simulink model "model"  (R2021a)
settings: Solver=VariableStepDiscrete  StartTime=0.0  StopTime=1000  RelTol=1e-3  EnableMultiTasking=on
PreLoadFcn:
  | initmod
values from neighbouring files (symbols this model uses):
  Bit_pat = Create_pat([1,0],1/(Ftr*2)-1/(2*Frc),1/Frc)    [initmod.m]
  Frc = Ftr*k    (= 16000)    [initmod.m]
  Ftr = 2000    [initmod.m]
  k = k+1    (= 2)    [initmod.m]
  pack_len = 11    [initmod.m]
  Preamble = [1,1,0,1,1,0,0,1,1,1,0,0,0,0,1,0]    [initmod.m]
  Preamble_decis_levl = ((Preamble_pat_len-Manchester_crosscorrelation*k/2)/2+Preamble_pat_len/2+Preamble_pat_len)/2-3    [initmod.m]
  Preamble_pat = Create_pat(Preamble,1/(Ftr*2),1/Frc)    [initmod.m]
  Preamble_pat_len = length(Preamble_pat)    [initmod.m]
undefined symbols (not defined in the file or in its folder): Bit_pat_len
libraries: dspobslib x14, dspswit3 x9, dspsigops x5, commutil2 x4, dspindex x4, commrandsrc3 x2, simulink_extras x1, commrandsrc2 x1, dspstat3 x1, commsink2 x1
settings Model: Creator=DeveloperY  LastModifiedBy=DeveloperY
settings DataIOCC: InitialState=init  LimitDataPoints=on  SaveFormat=Array  SignalLoggingSaveFormat=ModelDataLogs  ReturnWorkspaceOutputs=off
settings OptimizationCC: BlockReduction=off  BooleanDataType=off  OptimizeBlockIOStorage=off  BufferReuse=off  ExpressionFolding=off  LocalBlockOutputs=off  InitFltsAndDblsToZero=on  LifeSpan=inf
settings DebuggingCC: SaveWithParameterizedLinksMsg=none  UnderspecifiedInitializationDetection=Classic  MergeDetectMultiDrivingBlocksExec=none  SignalResolutionControl=TryResolveAllWithWarning  MultiTaskDSMMsg=warning  MultiTaskCondExecSysMsg=none  FcnCallInpInsideContextMsg=warning  SFUnexpectedBacktrackingDiag=warning  SFNoUnconditionalDefaultTransitionDiag=warning  SFExecutionAtInitializationDiag=none  SFMachineParentedDataDiag=warning  ArithmeticOperatorsInVariantConditions=warning
settings HardwareCC: ProdBitPerPointer=32  ProdBitPerSizeT=32  ProdBitPerPtrDiffT=32  ProdLargestAtomicFloat=None  ProdIntDivRoundTo=Undefined  ProdEndianess=Unspecified  ProdWordSize=32  ProdHWDeviceType=32-bit Generic  TargetUnknown=on
settings ModelReferenceCC: PropagateSignalLabelsOutOfModel=off
settings RTWCC: Description=Generic Real-Time Target
settings CodeAppCC: StateflowObjectComments=on
settings GRTTargetCC: TargetFcnLib=ansi_tfl_tmw.mat  TargetLangStandard=C89/C90 (ANSI)  CombineOutputUpdateFcns=off  GRTInterface=on
settings ConfigComp: CovMetricSettings=dw  CovSaveCumulativeToWorkspaceVar=on  CovSaveSingleToWorkspaceVar=on

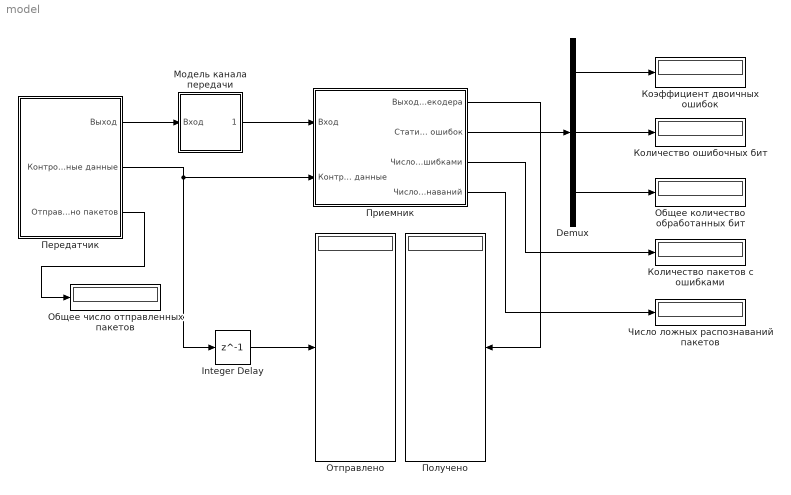
== system model ==
  Demux : Demux  Outputs=3
      settings: DisplayOption=none
  Integer Delay : Delay  DelayLength=1
  Количество ошибочных бит : Display
  Количество пакетов с ошибками : Display
  Коэффициент двоичных ошибок : Display
  Модель канала передачи : Subsystem  TreatAsAtomicUnit=on
  Общее количество обработанных бит : Display
  Общее число отправленных пакетов : Display
  Отправлено : Display
  Передатчик : Subsystem  TreatAsAtomicUnit=on
  Получено : Display
  Приемник : Subsystem  TreatAsAtomicUnit=on
  Число ложных распознаваний пакетов : Display
  wires:
  Передатчик/2(Контрольные данные) -> Приемник/2(Контрольные данные), Integer Delay/1
  Приемник/1(Выход декодера) -> Получено/1
  Приемник/2(Статистика ошибок) -> Demux/1
  Demux/1 -> Коэффициент двоичных ошибок/1
  Demux/2 -> Количество ошибочных бит/1
  Demux/3 -> Общее количество обработанных бит/1
  Приемник/3(Число пакетов с ошибками) -> Количество пакетов с ошибками/1
  Integer Delay/1 -> Отправлено/1
  Передатчик/1(Выход) -> Модель канала передачи/1(Вход)
  Модель канала передачи/1(Выход) -> Приемник/1("Вход ")
  Приемник/4(Число ложных распознаваний) -> Число ложных распознаваний пакетов/1
  Передатчик/3(Отправлено пакетов) -> Общее число отправленных пакетов/1

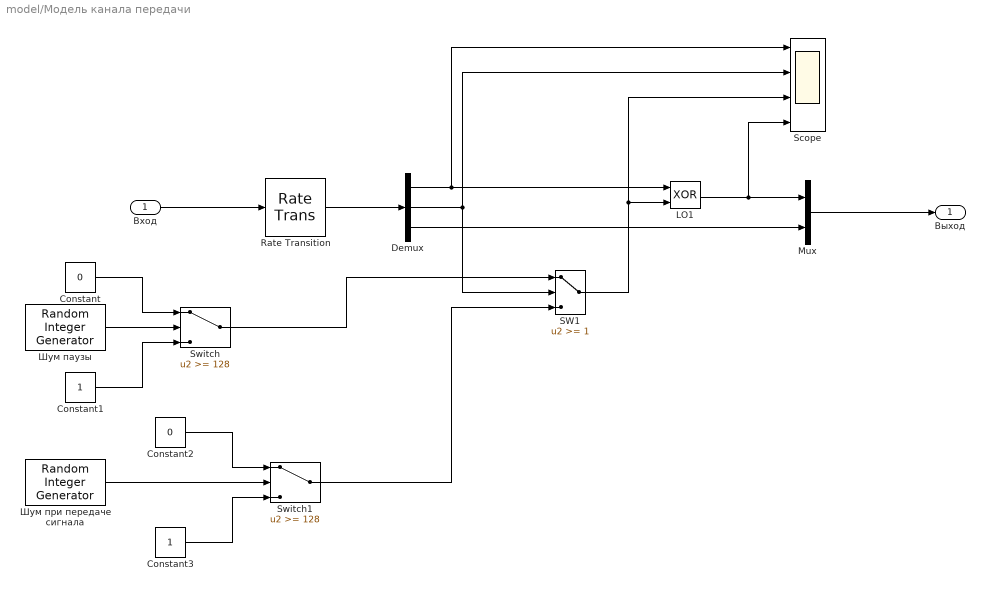
== system model/Модель канала передачи ==
  Вход : Inport
  Constant : Constant  Value=0
  Constant1 : Constant
  Constant2 : Constant  Value=0
  Constant3 : Constant
  Demux : Demux  Outputs=3
      settings: DisplayOption=none
  LO1 : Logic  Operator=XOR
  Mux : Mux  Inputs=2
  Rate Transition : RateTransition  Deterministic=off  OutPortSampleTime=1/Frc
  SW1 : Switch  Threshold=1  SaturateOnIntegerOverflow=on  InputSameDT=on
  Scope : Scope  NumInputPorts=4
  Switch : Switch  Threshold=128
  Switch1 : Switch  Threshold=128
  Шум паузы : commrandsrc3/Random Integer Generator  SetSize=1024  SeedSource=Auto  Seed=0  SampleTime=1/Frc  SamplesPerFrame=1  OutputDataType=double  SimulateUsing=Interpreted execution
  Шум при передаче сигнала : commrandsrc3/Random Integer Generator  SetSize=1024  SeedSource=Auto  Seed=0  SampleTime=1/Frc  SamplesPerFrame=1  OutputDataType=double  SimulateUsing=Interpreted execution
  Выход : Outport
  wires:
  Rate Transition/1 -> Demux/1
  Demux/2 -> Scope/2, SW1/2
  SW1/1 -> Scope/3, LO1/2
  Demux/1 -> Scope/1, LO1/1
  Шум при передаче сигнала/1 -> Switch1/2
  Шум паузы/1 -> Switch/2
  Вход/1 -> Rate Transition/1
  LO1/1 -> Scope/4, Mux/1
  Mux/1 -> Выход/1
  Demux/3 -> Mux/2
  Switch1/1 -> SW1/3
  Constant/1 -> Switch/1
  Constant1/1 -> Switch/3
  Switch/1 -> SW1/1
  Constant3/1 -> Switch1/3
  Constant2/1 -> Switch1/1

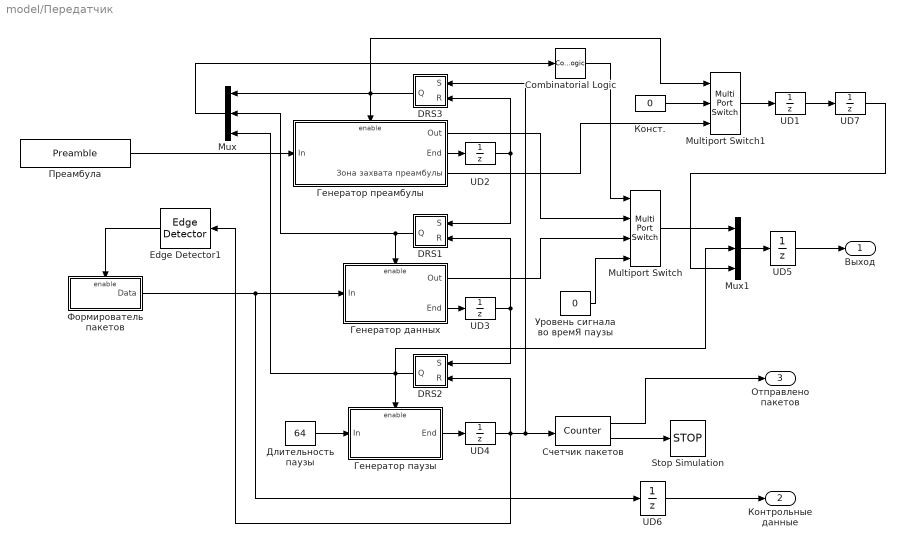
== system model/Передатчик ==
  Combinatorial Logic : CombinatorialLogic  TruthTable=[1;3;2;2;1;1;1;1]
  DRS1 : Subsystem  TreatAsAtomicUnit=on
  DRS2 : Subsystem  TreatAsAtomicUnit=on
  DRS3 : Subsystem  TreatAsAtomicUnit=on
  Edge Detector1 : dspswit3/Edge Detector  InputProcessing=Columns as channels (frame based)
      settings: SourceProductBaseCode=DS
  Multiport Switch : MultiPortSwitch  SaturateOnIntegerOverflow=on  InputSameDT=on
  Multiport Switch1 : MultiPortSwitch  DataPortOrder=Zero-based contiguous  Inputs=2  zeroidx=on  SaturateOnIntegerOverflow=on  InputSameDT=on
  Mux : Mux  Inputs=3
  Mux1 : Mux  Inputs=3
  Stop Simulation : Stop
  UD{1..2,4,7} (4 alike) : UnitDelay  SampleTime=-1
  UD3 : UnitDelay  InitialCondition=1  SampleTime=-1
  UD5 : UnitDelay  SampleTime=1/(Ftr*4)
  UD6 : UnitDelay  SampleTime=1/(Ftr*4)
  Генератор данных : Subsystem  TreatAsAtomicUnit=on
  Генератор паузы : Subsystem  TreatAsAtomicUnit=on
  Генератор преамбулы : Subsystem  TreatAsAtomicUnit=on
  Длительность паузы : Constant  Value=64
  Конст. : Constant  Value=0
  Преамбула : Constant  Value=Preamble
  Счетчик пакетов : dspswit3/Counter  Direction=Up  CountEvent=Rising edge  CounterSize=User defined  MaxCount=pack_num  InitialCount=0  Output=Count and Hit  HitValue=pack_num  ResetInput=off  SamplesPerFrame=1  Ts=1  CntDtype=double  HitDtype=Logical
  Уровень сигнала во времЯ паузы : Constant  Value=0
  Формирователь пакетов : Subsystem  TreatAsAtomicUnit=on
  Выход : Outport
  Контрольные данные : Outport  Port=2
  Отправлено пакетов : Outport  Port=3
  wires:
  Преамбула/1 -> Генератор преамбулы/1(In)
  Multiport Switch/1 -> Mux1/1
  Генератор преамбулы/1(Out) -> Multiport Switch/2
  Длительность паузы/1 -> Генератор паузы/1(In)
  Генератор данных/2(End) -> UD3/1
  Генератор преамбулы/2(End) -> UD2/1
  UD3/1 -> DRS1/2(R), DRS2/1(S)
  UD2/1 -> DRS1/1(S), DRS3/2(R)
  DRS1/1(Q) -> Генератор данных/Enable, Mux/2
  DRS3/1(Q) -> Генератор преамбулы/Enable, Mux/1, Multiport Switch1/1
  Генератор паузы/1(End) -> UD4/1
  UD4/1 -> DRS3/1(S), Счетчик пакетов/1, DRS2/2(R), Edge Detector1/1
  DRS2/1(Q) -> Mux/3, Генератор паузы/Enable, Mux1/2
  Combinatorial Logic/1 -> Multiport Switch/1
  Генератор данных/1(Out) -> Multiport Switch/3
  Mux/1 -> Combinatorial Logic/1
  Уровень сигнала во времЯ паузы/1 -> Multiport Switch/4
  Mux1/1 -> UD5/1
  UD5/1 -> Выход/1
  UD6/1 -> Контрольные данные/1
  Формирователь пакетов/1(Data) -> Генератор данных/1(In), UD6/1
  Edge Detector1/1 -> Формирователь пакетов/Enable
  Счетчик пакетов/1 -> Отправлено пакетов/1
  Конст./1 -> Multiport Switch1/2
  Генератор преамбулы/3(Зона захвата преамбулы) -> Multiport Switch1/3
  Multiport Switch1/1 -> UD1/1
  UD1/1 -> UD7/1
  UD7/1 -> Mux1/3
  Счетчик пакетов/2 -> Stop Simulation/1

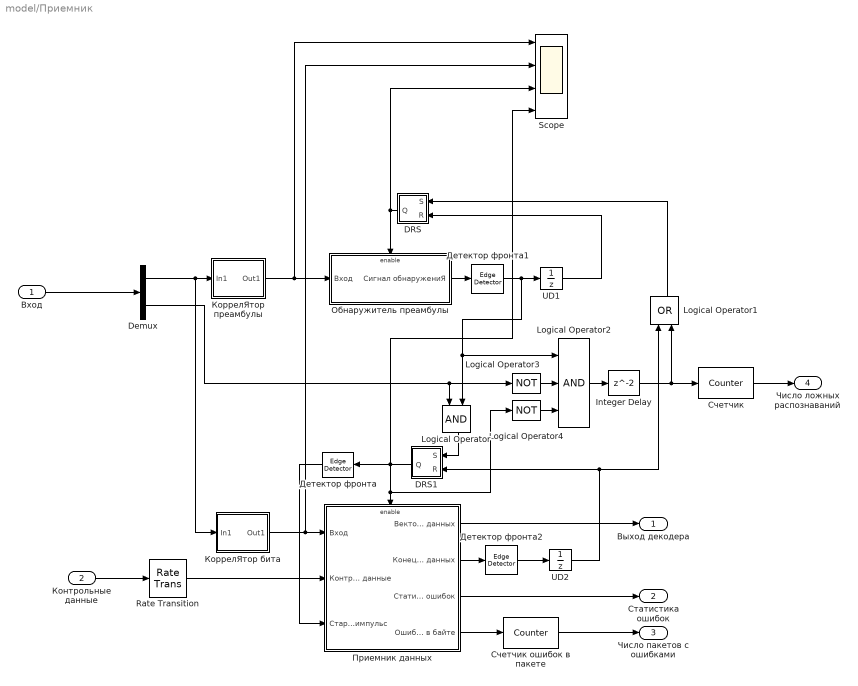
== system model/Приемник ==
  "Вход " : Inport
  Контрольные данные : Inport  Port=2
  " КоррелЯтор преамбулы" : Subsystem  TreatAsAtomicUnit=on
  " КоррелЯтор бита" : Subsystem  TreatAsAtomicUnit=on
  DRS : Subsystem  TreatAsAtomicUnit=on
  DRS1 : Subsystem  TreatAsAtomicUnit=on
  Demux : Demux  Outputs=2
  Integer Delay : Delay
  Logical Operator : Logic  AllPortsSameDT=off
  Logical Operator1 : Logic  Operator=OR  AllPortsSameDT=off
  Logical Operator2 : Logic  Inputs=3  AllPortsSameDT=off
  Logical Operator3 : Logic  Operator=NOT  Inputs=1  AllPortsSameDT=off  OutDataTypeStr=boolean
  Logical Operator4 : Logic  Operator=NOT  Inputs=1  AllPortsSameDT=off  OutDataTypeStr=boolean
  Rate Transition : RateTransition  Deterministic=off  OutPortSampleTime=1/Frc
  Scope : Scope  NumInputPorts=4
  UD1 : UnitDelay  SampleTime=-1
  UD2 : UnitDelay  InitialCondition=1  SampleTime=-1
  Детектор фронта : dspswit3/Edge Detector  InputProcessing=Columns as channels (frame based)
      settings: SourceProductBaseCode=DS
  Детектор фронта1 : dspswit3/Edge Detector  InputProcessing=Columns as channels (frame based)
      settings: SourceProductBaseCode=DS
  Детектор фронта2 : dspswit3/Edge Detector  InputProcessing=Columns as channels (frame based)
      settings: SourceProductBaseCode=DS
  Обнаружитель преамбулы : Subsystem  TreatAsAtomicUnit=on
  Приемник данных : Subsystem  TreatAsAtomicUnit=on
  "Счетчик " : dspswit3/Counter  Direction=Up  CountEvent=Rising edge  CounterSize=32 bits  MaxCount=255  InitialCount=0  Output=Count  HitValue=32  ResetInput=off  SamplesPerFrame=1  Ts=1  CntDtype=uint32  HitDtype=Logical
  Счетчик ошибок в пакете : dspswit3/Counter  Direction=Up  CountEvent=Falling edge  CounterSize=32 bits  MaxCount=255  InitialCount=0  Output=Count  HitValue=32  ResetInput=off  SamplesPerFrame=1  Ts=1  CntDtype=double  HitDtype=Logical
  Выход декодера : Outport
  Статистика ошибок : Outport  Port=2
  Число пакетов с ошибками : Outport  Port=3
  Число ложных распознаваний : Outport  Port=4
  wires:
  Приемник данных/1(Вектор выходных данных) -> Выход декодера/1
  Приемник данных/3(Статистика ошибок) -> Статистика ошибок/1
  DRS/1(Q) -> Обнаружитель преамбулы/Enable, Scope/3
  DRS1/1(Q) -> Scope/4, Детектор фронта/1, Приемник данных/Enable, Logical Operator4/1
  UD1/1 -> DRS/2(R)
  Обнаружитель преамбулы/1(Сигнал обнаружениЯ) -> Детектор фронта1/1
  Приемник данных/2(Конец блока данных) -> Детектор фронта2/1
  UD2/1 -> DRS1/2(R), Logical Operator1/1
  Приемник данных/4(Ошибка в байте) -> Счетчик ошибок в пакете/1
  " КоррелЯтор бита"/1(Out1) -> Scope/2, Приемник данных/1(Вход)
  " КоррелЯтор преамбулы"/1(Out1) -> Scope/1, Обнаружитель преамбулы/1(Вход)
  Детектор фронта/1 -> Приемник данных/3(Старт. импульс)
  Счетчик ошибок в пакете/1 -> Число пакетов с ошибками/1
  Контрольные данные/1 -> Rate Transition/1
  Rate Transition/1 -> Приемник данных/2(Контрольные данные)
  "Вход "/1 -> Demux/1
  Demux/1 -> " КоррелЯтор преамбулы"/1(In1), " КоррелЯтор бита"/1(In1)
  Demux/2 -> Logical Operator/1, Logical Operator3/1
  Logical Operator/1 -> DRS1/1(S)
  Logical Operator1/1 -> DRS/1(S)
  Logical Operator3/1 -> Logical Operator2/2
  Logical Operator2/1 -> Integer Delay/1
  "Счетчик "/1 -> Число ложных распознаваний/1
  Integer Delay/1 -> "Счетчик "/1, Logical Operator1/2
  Детектор фронта1/1 -> UD1/1, Logical Operator/2, Logical Operator2/1
  Детектор фронта2/1 -> UD2/1
  Logical Operator4/1 -> Logical Operator2/3

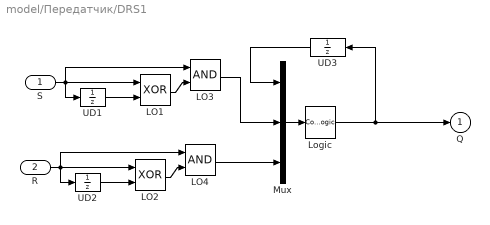
== system model/Передатчик/DRS1 ==
  S : Inport
  R : Inport  Port=2
  LO1 : Logic  Operator=XOR
  LO2 : Logic  Operator=XOR
  LO3 : Logic
  LO4 : Logic
  Logic : CombinatorialLogic  TruthTable=[0 ;0 ;1 ;0 ;1 ;0 ;1 ;1 ]
  Mux : Mux  Inputs=3
  UD1 : UnitDelay  SampleTime=-1
  UD2 : UnitDelay  SampleTime=-1
  UD3 : UnitDelay  SampleTime=-1
  Q : Outport  InitialOutput=0
  wires:
  Mux/1 -> Logic/1
  UD3/1 -> Mux/1
  LO3/1 -> Mux/2
  LO4/1 -> Mux/3
  Logic/1 -> UD3/1, Q/1
  S/1 -> LO1/1, UD1/1, LO3/1
  UD1/1 -> LO1/2
  LO1/1 -> LO3/2
  R/1 -> LO2/1, UD2/1, LO4/1
  UD2/1 -> LO2/2
  LO2/1 -> LO4/2

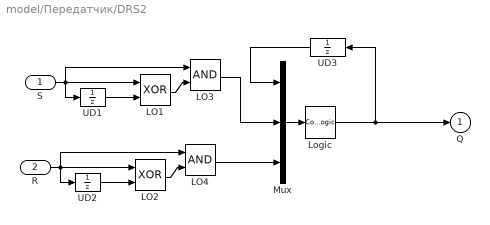
== system model/Передатчик/DRS2 ==
  S : Inport
  R : Inport  Port=2
  LO1 : Logic  Operator=XOR
  LO2 : Logic  Operator=XOR
  LO3 : Logic
  LO4 : Logic
  Logic : CombinatorialLogic  TruthTable=[0 ;0 ;1 ;0 ;1 ;0 ;1 ;1 ]
  Mux : Mux  Inputs=3
  UD1 : UnitDelay  SampleTime=-1
  UD2 : UnitDelay  SampleTime=-1
  UD3 : UnitDelay  SampleTime=-1
  Q : Outport  InitialOutput=0
  wires:
  Mux/1 -> Logic/1
  UD3/1 -> Mux/1
  LO3/1 -> Mux/2
  LO4/1 -> Mux/3
  Logic/1 -> UD3/1, Q/1
  S/1 -> LO1/1, UD1/1, LO3/1
  UD1/1 -> LO1/2
  LO1/1 -> LO3/2
  R/1 -> LO2/1, UD2/1, LO4/1
  UD2/1 -> LO2/2
  LO2/1 -> LO4/2

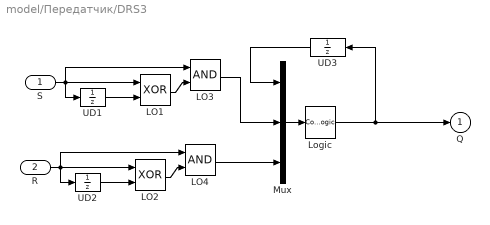
== system model/Передатчик/DRS3 ==
  S : Inport
  R : Inport  Port=2
  LO1 : Logic  Operator=XOR
  LO2 : Logic  Operator=XOR
  LO3 : Logic
  LO4 : Logic
  Logic : CombinatorialLogic  TruthTable=[0 ;0 ;1 ;0 ;1 ;0 ;1 ;1 ]
  Mux : Mux  Inputs=3
  UD1 : UnitDelay  SampleTime=-1
  UD2 : UnitDelay  SampleTime=-1
  UD3 : UnitDelay  SampleTime=-1
  Q : Outport  InitialOutput=0
  wires:
  Mux/1 -> Logic/1
  UD3/1 -> Mux/1
  LO3/1 -> Mux/2
  LO4/1 -> Mux/3
  Logic/1 -> UD3/1, Q/1
  S/1 -> LO1/1, UD1/1, LO3/1
  UD1/1 -> LO1/2
  LO1/1 -> LO3/2
  R/1 -> LO2/1, UD2/1, LO4/1
  UD2/1 -> LO2/2
  LO2/1 -> LO4/2

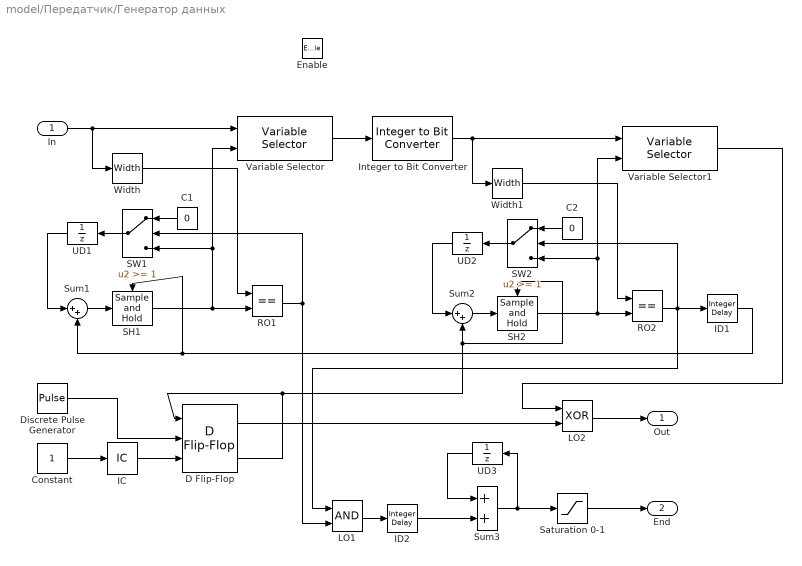
== system model/Передатчик/Генератор данных ==
  In : Inport
  Enable : EnablePort  StatesWhenEnabling=reset
  C1 : Constant  Value=0
  C2 : Constant  Value=0
  Constant : Constant
  D Flip-Flop : simulink_extras/Flip Flops/D Flip-Flop
  Discrete Pulse Generator : DiscretePulseGenerator  SampleTime=1/(Ftr*4)
  IC : InitialCondition  Value=0
  ID1 : dspobslib/Integer Delay  delay=4  ic=1  reset_popup=None
      settings: SourceProductBaseCode=DS
  ID2 : dspobslib/Integer Delay  delay=4-1  ic=0  reset_popup=None
      settings: SourceProductBaseCode=DS
  Integer to Bit Converter : commutil2/Integer to Bit Converter  nbits=8  signedInputValues=Unsigned  bitOrder=MSB first  outDtype=Inherit via internal rule
  LO1 : Logic
  LO2 : Logic  Operator=XOR
  RO1 : RelationalOperator  Operator===  RndMeth=Nearest  InputSameDT=on
  RO2 : RelationalOperator  Operator===  RndMeth=Nearest  InputSameDT=on
  SH1 : dspsigops/Sample and Hold  trig=Rising edge  initCond=1  latchinput=off
  SH2 : dspsigops/Sample and Hold  trig=Rising edge  initCond=1  latchinput=off
  SW1 : Switch  Threshold=1  SaturateOnIntegerOverflow=on  InputSameDT=on
  SW2 : Switch  Threshold=1  SaturateOnIntegerOverflow=on  InputSameDT=on
  Saturation 0-1 : Saturate  UpperLimit=1  LowerLimit=0
  Sum1 : Sum  Inputs=|++  InputSameDT=on  SaturateOnIntegerOverflow=on  OutDataTypeStr=Inherit: Same as first input
  Sum2 : Sum  Inputs=|++  InputSameDT=on  SaturateOnIntegerOverflow=on  OutDataTypeStr=Inherit: Same as first input
  Sum3 : Sum  InputSameDT=on  SaturateOnIntegerOverflow=on  OutDataTypeStr=Inherit: Same as first input
  UD1 : UnitDelay  SampleTime=-1
  UD2 : UnitDelay  SampleTime=-1
  UD3 : UnitDelay  SampleTime=-1
  Variable Selector : dspindex/Variable Selector  NumInputs=1  rowsOrCols=Columns  IdxMode=Variable  Elements=[1 3]  ZerOneIdxMode=One-based  errmode=Clip Index  FillMode=on  FillValues=0
  Variable Selector1 : dspindex/Variable Selector  NumInputs=1  rowsOrCols=Columns  IdxMode=Variable  Elements=[1 3]  ZerOneIdxMode=One-based  errmode=Clip Index  FillMode=on  FillValues=0
  Width : Width
  Width1 : Width
  Out : Outport  InitialOutput=[0]
  End : Outport  Port=2  InitialOutput=[0]
  wires:
  Variable Selector/1 -> Integer to Bit Converter/1
  Integer to Bit Converter/1 -> Variable Selector1/1, Width1/1
  In/1 -> Variable Selector/1, Width/1
  UD1/1 -> Sum1/1
  RO1/1 -> SW1/2, LO1/2
  SW1/1 -> UD1/1
  C1/1 -> SW1/1
  Width/1 -> RO1/1
  Sum1/1 -> SH1/1
  UD2/1 -> Sum2/1
  RO2/1 -> SW2/2, ID1/1, LO1/1
  SW2/1 -> UD2/1
  C2/1 -> SW2/1
  Width1/1 -> RO2/1
  Sum2/1 -> SH2/1
  ID1/1 -> SH1/Trigger, Sum1/2
  Variable Selector1/1 -> LO2/1
  Discrete Pulse Generator/1 -> D Flip-Flop/2
  LO2/1 -> Out/1
  D Flip-Flop/1 -> LO2/2
  Sum3/1 -> UD3/1, Saturation 0-1/1
  LO1/1 -> ID2/1
  ID2/1 -> Sum3/2
  Saturation 0-1/1 -> End/1
  UD3/1 -> Sum3/1
  SH1/1 -> RO1/2, Variable Selector/2, SW1/3
  SH2/1 -> RO2/2, Variable Selector1/2, SW2/3
  D Flip-Flop/2 -> SH2/Trigger, Sum2/2, D Flip-Flop/1
  Constant/1 -> IC/1
  IC/1 -> D Flip-Flop/3

== system model/Передатчик/Генератор паузы ==
  In : Inport
  Enable : EnablePort  StatesWhenEnabling=reset
  Constant1 : Constant
  Constant3 : Constant  Value=0
  Relational Operator2 : RelationalOperator  Operator===  RndMeth=Nearest  InputSameDT=on
  Sum1 : Sum  Inputs=|++  InputSameDT=on  SaturateOnIntegerOverflow=on  OutDataTypeStr=Inherit: Same as first input
  Switch3 : Switch  Threshold=1  SaturateOnIntegerOverflow=on  InputSameDT=on
  Unit Delay3 : UnitDelay  SampleTime=-1
  End : Outport  InitialOutput=[0]
  wires:
  Unit Delay3/1 -> Sum1/1
  Relational Operator2/1 -> Switch3/2, End/1
  Switch3/1 -> Unit Delay3/1
  Constant3/1 -> Switch3/1
  In/1 -> Relational Operator2/1
  Sum1/1 -> Relational Operator2/2, Switch3/3
  Constant1/1 -> Sum1/2

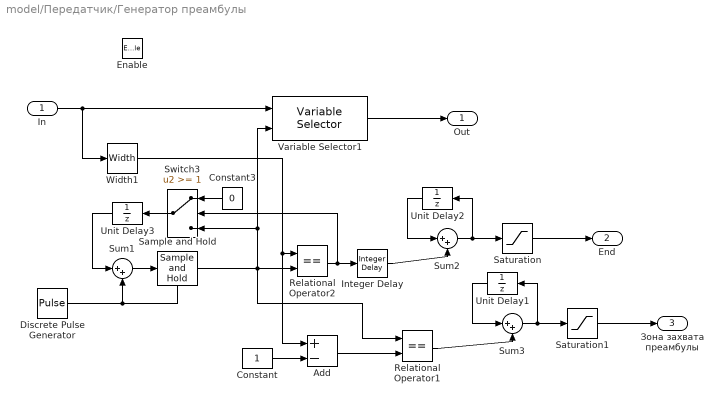
== system model/Передатчик/Генератор преамбулы ==
  In : Inport
  Enable : EnablePort  StatesWhenEnabling=reset
  Add : Sum  Inputs=+-
  Constant : Constant
  Constant3 : Constant  Value=0
  Discrete Pulse Generator : DiscretePulseGenerator  SampleTime=1/(Ftr*4)
  Integer Delay : dspobslib/Integer Delay  delay=2-1  ic=0  reset_popup=None
      settings: SourceProductBaseCode=DS
  Relational Operator1 : RelationalOperator  Operator===  RndMeth=Nearest  InputSameDT=on
  Relational Operator2 : RelationalOperator  Operator===  RndMeth=Nearest  InputSameDT=on
  Sample and Hold : dspsigops/Sample and Hold  trig=Rising edge  initCond=1  latchinput=off
  Saturation : Saturate  UpperLimit=1  LowerLimit=0
  Saturation1 : Saturate  UpperLimit=1  LowerLimit=0
  Sum1 : Sum  Inputs=|++  InputSameDT=on  SaturateOnIntegerOverflow=on  OutDataTypeStr=Inherit: Same as first input
  Sum2 : Sum  Inputs=|++  InputSameDT=on  SaturateOnIntegerOverflow=on  OutDataTypeStr=Inherit: Same as first input
  Sum3 : Sum  Inputs=|++  InputSameDT=on  SaturateOnIntegerOverflow=on  OutDataTypeStr=Inherit: Same as first input
  Switch3 : Switch  Threshold=1  SaturateOnIntegerOverflow=on  InputSameDT=on
  Unit Delay1 : UnitDelay  SampleTime=-1
  Unit Delay2 : UnitDelay  SampleTime=-1
  Unit Delay3 : UnitDelay  SampleTime=-1
  Variable Selector1 : dspindex/Variable Selector  NumInputs=1  rowsOrCols=Columns  IdxMode=Variable  Elements=[1 3]  ZerOneIdxMode=One-based  errmode=Clip Index  FillMode=on  FillValues=0
  Width1 : Width
  Out : Outport  InitialOutput=[0]
  End : Outport  Port=2  InitialOutput=[0]
  Зона захвата преамбулы : Outport  Port=3  InitialOutput=[0]
  wires:
  In/1 -> Variable Selector1/1, Width1/1
  Variable Selector1/1 -> Out/1
  Unit Delay3/1 -> Sum1/1
  Relational Operator2/1 -> Switch3/2, Integer Delay/1
  Switch3/1 -> Unit Delay3/1
  Constant3/1 -> Switch3/1
  Integer Delay/1 -> Sum2/2
  Width1/1 -> Relational Operator2/1, Add/1
  Discrete Pulse Generator/1 -> Sum1/2, Sample and Hold/Trigger
  Sum1/1 -> Sample and Hold/1
  Sample and Hold/1 -> Relational Operator2/2, Variable Selector1/2, Switch3/3, Relational Operator1/1
  Sum2/1 -> Unit Delay2/1, Saturation/1
  Unit Delay2/1 -> Sum2/1
  Saturation/1 -> End/1
  Constant/1 -> Add/2
  Add/1 -> Relational Operator1/2
  Sum3/1 -> Unit Delay1/1, Saturation1/1
  Saturation1/1 -> Зона захвата преамбулы/1
  Unit Delay1/1 -> Sum3/1
  Relational Operator1/1 -> Sum3/2

== system model/Передатчик/Формирователь пакетов ==
  Enable : EnablePort
  Constant : Constant  Value=repmat(17,1,pack_len)  OutDataTypeStr=uint8
  Frame Status Conversion : dspobslib/Frame Status Conversion  growRefPort=off  outframe=Sample-based
      settings: SourceProductBaseCode=DS
  Manual Switch : ManualSwitch
  Random-Integer Generator : commrandsrc2/Random Integer Generator  mul=256  seed=[12345]  Ts=1/(Ftr*4*pack_len)  frameBased=on  sampPerFrame=pack_len  orient=off  outDataType=double
      settings: SourceProductBaseCode=CM
  Reshape : Reshape
  Data : Outport
  wires:
  Random-Integer Generator/1 -> Frame Status Conversion/1
  Reshape/1 -> Data/1
  Manual Switch/1 -> Reshape/1
  Frame Status Conversion/1 -> Manual Switch/1
  Constant/1 -> Manual Switch/2

== system model/Приемник/ КоррелЯтор преамбулы ==
  In1 : Inport
  Buffer : Buffer  N=Preamble_pat_len  V=Preamble_pat_len-1
  Frame Status Conversion : dspobslib/Frame Status Conversion  growRefPort=off  outframe=Sample-based
      settings: SourceProductBaseCode=DS
  Logical Operator : Logic  Operator=XOR
  Logical Operator1 : Logic  Operator=NOT
  Matrix Sum : dspobslib/Matrix Sum  Dim=Columns  roundingMode=Floor  overflowMode=off
      settings: SourceProductBaseCode=DS
  Шаблон преамбулы : dspobslib/DSP Constant  Value=Preamble_pat  SampleMode=Discrete  discreteOutput=Frame-based  continuousOutput=Sample-based  sampTime=-1  framePeriod=-1  dataType=Inherit from 'Constant value'  isSigned=on  wordLen=16  udDataType=sfix(16)  fracBitsMode=Best precision  numFracBits=15  InterpretAs1D=off  Ts=-1  FramebasedOutput=on
      settings: SourceProductBaseCode=DS
  Out1 : Outport
  wires:
  In1/1 -> Buffer/1
  Matrix Sum/1 -> Out1/1
  Frame Status Conversion/1 -> Matrix Sum/1
  Buffer/1 -> Logical Operator/1
  Шаблон преамбулы/1 -> Logical Operator/2
  Logical Operator/1 -> Logical Operator1/1
  Logical Operator1/1 -> Frame Status Conversion/1

== system model/Приемник/ КоррелЯтор бита ==
  In1 : Inport
  Bit pattern : dspobslib/DSP Constant  Value=Bit_pat  SampleMode=Discrete  discreteOutput=Frame-based  continuousOutput=Sample-based  sampTime=-1  framePeriod=-1  dataType=Inherit from 'Constant value'  isSigned=on  wordLen=16  udDataType=sfix(16)  fracBitsMode=Best precision  numFracBits=15  InterpretAs1D=off  Ts=-1  FramebasedOutput=on
      settings: SourceProductBaseCode=DS
  Buffer1 : Buffer  N=Bit_pat_len  V=Bit_pat_len-1
  Frame Status Conversion1 : dspobslib/Frame Status Conversion  growRefPort=off  outframe=Sample-based
      settings: SourceProductBaseCode=DS
  Logical Operator3 : Logic  Operator=XOR
  Logical Operator4 : Logic  Operator=NOT
  Matrix Sum1 : dspobslib/Matrix Sum  Dim=Columns  roundingMode=Floor  overflowMode=off
      settings: SourceProductBaseCode=DS
  Out1 : Outport
  wires:
  In1/1 -> Buffer1/1
  Frame Status Conversion1/1 -> Matrix Sum1/1
  Buffer1/1 -> Logical Operator3/1
  Bit pattern/1 -> Logical Operator3/2
  Logical Operator3/1 -> Logical Operator4/1
  Logical Operator4/1 -> Frame Status Conversion1/1
  Matrix Sum1/1 -> Out1/1

== system model/Приемник/DRS ==
  S : Inport
  R : Inport  Port=2
  LO1 : Logic  Operator=XOR
  LO2 : Logic  Operator=XOR
  LO3 : Logic
  LO4 : Logic
  Logic : CombinatorialLogic  TruthTable=[0 ;0 ;1 ;0 ;1 ;0 ;1 ;1 ]
  Mux : Mux  Inputs=3
  UD1 : UnitDelay  SampleTime=-1
  UD2 : UnitDelay  SampleTime=-1
  UD3 : UnitDelay  SampleTime=-1
  Q : Outport  InitialOutput=0
  wires:
  Mux/1 -> Logic/1
  UD3/1 -> Mux/1
  LO3/1 -> Mux/2
  LO4/1 -> Mux/3
  Logic/1 -> UD3/1, Q/1
  S/1 -> LO1/1, UD1/1, LO3/1
  UD1/1 -> LO1/2
  LO1/1 -> LO3/2
  R/1 -> LO2/1, UD2/1, LO4/1
  UD2/1 -> LO2/2
  LO2/1 -> LO4/2

== system model/Приемник/DRS1 ==
  S : Inport
  R : Inport  Port=2
  LO1 : Logic  Operator=XOR
  LO2 : Logic  Operator=XOR
  LO3 : Logic
  LO4 : Logic
  Logic : CombinatorialLogic  TruthTable=[0 ;0 ;1 ;0 ;1 ;0 ;1 ;1 ]
  Mux : Mux  Inputs=3
  UD1 : UnitDelay  SampleTime=-1
  UD2 : UnitDelay  SampleTime=-1
  UD3 : UnitDelay  SampleTime=-1
  Q : Outport  InitialOutput=0
  wires:
  Mux/1 -> Logic/1
  UD3/1 -> Mux/1
  LO3/1 -> Mux/2
  LO4/1 -> Mux/3
  Logic/1 -> UD3/1, Q/1
  S/1 -> LO1/1, UD1/1, LO3/1
  UD1/1 -> LO1/2
  LO1/1 -> LO3/2
  R/1 -> LO2/1, UD2/1, LO4/1
  UD2/1 -> LO2/2
  LO2/1 -> LO4/2

== system model/Приемник/Обнаружитель преамбулы ==
  Вход : Inport
  Enable : EnablePort  StatesWhenEnabling=reset
  Logical Operator2 : Logic
  Maximum : dspstat3/Maximum  operation=maximum  fcn=Running  indexBase=One  operateOver=Each column  Dimension=1  InputProcessing=Columns as channels (frame based)  reset=Rising edge  roiEnable=off  roiType=Rectangles  roiPortion=Entire ROI  roiOutput=Individual statistics for each ROI  roiFlag=off  roundingMode=Floor  overflowMode=off  accumDataTypeStr=Inherit: Same as product output  accumLastDataTypeStr=Inherit: Same as product output
  RO1 : RelationalOperator  Operator=>  RndMeth=Nearest  InputSameDT=on
  Relational Operator : RelationalOperator  RndMeth=Nearest  InputSameDT=on
  UD1 : UnitDelay  SampleTime=-1
  Уровень обнаружениЯ : Constant  Value=Preamble_decis_levl
  Сигнал обнаружениЯ : Outport  InitialOutput=[0]
  wires:
  Вход/1 -> Maximum/1, RO1/2
  Maximum/1 -> Relational Operator/1, RO1/1
  RO1/1 -> Logical Operator2/2, UD1/1
  Relational Operator/1 -> Logical Operator2/1
  UD1/1 -> Maximum/2
  Уровень обнаружениЯ/1 -> Relational Operator/2
  Logical Operator2/1 -> Сигнал обнаружениЯ/1

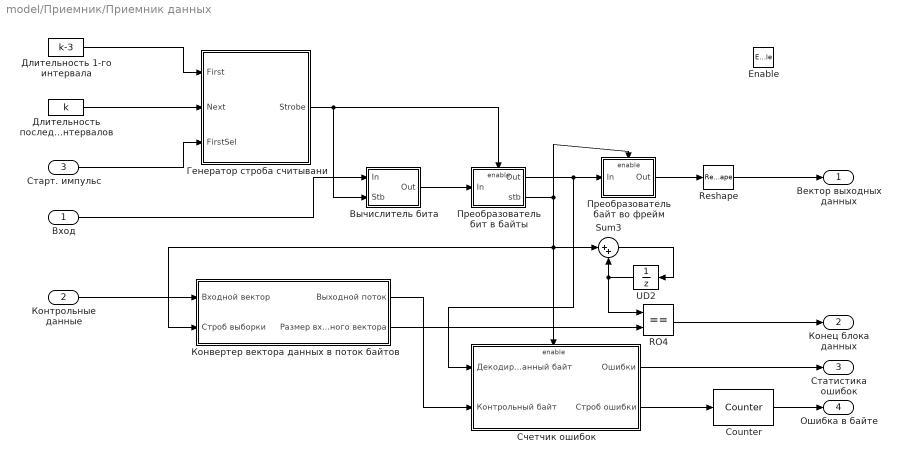
== system model/Приемник/Приемник данных ==
  Вход : Inport
  Контрольные данные : Inport  Port=2
  Старт. импульс : Inport  Port=3
  Enable : EnablePort  StatesWhenEnabling=reset
  Counter : dspswit3/Counter  Direction=Up  CountEvent=Rising edge  CounterSize=32 bits  MaxCount=255  InitialCount=0  Output=Count  HitValue=32  ResetInput=off  SamplesPerFrame=1  Ts=1  CntDtype=double  HitDtype=Logical
  RO4 : RelationalOperator  Operator===  RndMeth=Nearest  InputSameDT=on
  Reshape : Reshape
  Sum3 : Sum  Inputs=|++  InputSameDT=on  SaturateOnIntegerOverflow=on  OutDataTypeStr=Inherit: Same as first input
  UD2 : UnitDelay  SampleTime=-1
  Вычислитель бита : Subsystem  TreatAsAtomicUnit=on
  Генератор строба считывани : Subsystem
  Длительность 1-го интервала : Constant  Value=k-3
  Длительность последующих интервалов : Constant  Value=k
  Конвертер вектора данных в поток байтов : Subsystem  TreatAsAtomicUnit=on
  Преобразователь байт во фрейм : Subsystem  TreatAsAtomicUnit=on
  Преобразователь бит в байты : Subsystem  TreatAsAtomicUnit=on
  Счетчик ошибок : Subsystem  TreatAsAtomicUnit=on
  Вектор выходных данных : Outport  InitialOutput=[0]
  Конец блока данных : Outport  Port=2  InitialOutput=[0]
  Статистика ошибок : Outport  Port=3  InitialOutput=[0]
  Ошибка в байте : Outport  Port=4  OutputWhenDisabled=reset  InitialOutput=[0]
  wires:
  Вход/1 -> Вычислитель бита/1(In)
  Длительность 1-го интервала/1 -> Генератор строба считывани/1(First)
  Преобразователь бит в байты/1(Out) -> Преобразователь байт во фрейм/1(In), Счетчик ошибок/1(Декодированный байт)
  Преобразователь бит в байты/2(stb) -> Sum3/1, Счетчик ошибок/Enable, Конвертер вектора данных в поток байтов/2(Строб выборки), Преобразователь байт во фрейм/Enable
  RO4/1 -> Конец блока данных/1
  Sum3/1 -> UD2/1
  UD2/1 -> RO4/1, Sum3/2
  Вычислитель бита/1(Out) -> Преобразователь бит в байты/1(In)
  Генератор строба считывани/1(Strobe) -> Вычислитель бита/2(Stb), Преобразователь бит в байты/Enable
  Преобразователь байт во фрейм/1(Out) -> Reshape/1
  Reshape/1 -> Вектор выходных данных/1
  Счетчик ошибок/1(Ошибки) -> Статистика ошибок/1
  Счетчик ошибок/2(Строб ошибки) -> Counter/1
  Counter/1 -> Ошибка в байте/1
  Длительность последующих интервалов/1 -> Генератор строба считывани/2(Next)
  Старт. импульс/1 -> Генератор строба считывани/3(FirstSel)
  Контрольные данные/1 -> Конвертер вектора данных в поток байтов/1(Входной вектор)
  Конвертер вектора данных в поток байтов/1(Выходной поток) -> Счетчик ошибок/2(Контрольный байт)
  Конвертер вектора данных в поток байтов/2(Размер входного вектора) -> RO4/2

== system model/Приемник/Приемник данных/Вычислитель бита ==
  In : Inport
  Stb : Inport  Port=2
  Constant : Constant
  Constant1 : Constant  Value=0
  Constant7 : Constant  Value=k/2-1
  Gain1 : Gain  Gain=2  SaturateOnIntegerOverflow=on  OutDataTypeStr=Inherit: Same as input  ParamDataTypeStr=Inherit: Same as input
  Multiport Switch : MultiPortSwitch  Inputs=2  SaturateOnIntegerOverflow=on  InputSameDT=on
  Relational Operator2 : RelationalOperator  Operator=<=  RndMeth=Nearest  InputSameDT=on
  Relational Operator3 : RelationalOperator  Operator=>  RndMeth=Nearest  InputSameDT=on
  Sample and Hold1 : dspsigops/Sample and Hold  trig=Rising edge  initCond=0  latchinput=off
  Sum1 : Sum  InputSameDT=on  SaturateOnIntegerOverflow=on  OutDataTypeStr=Inherit: Same as first input
  Out : Outport
  wires:
  In/1 -> Relational Operator3/1, Relational Operator2/1
  Constant7/1 -> Relational Operator3/2, Relational Operator2/2
  Relational Operator2/1 -> Gain1/1
  Relational Operator3/1 -> Sum1/1
  Sum1/1 -> Multiport Switch/1
  Constant/1 -> Multiport Switch/2
  Constant1/1 -> Multiport Switch/3
  Multiport Switch/1 -> Sample and Hold1/1
  Sample and Hold1/1 -> Out/1
  Stb/1 -> Sample and Hold1/Trigger
  Gain1/1 -> Sum1/2

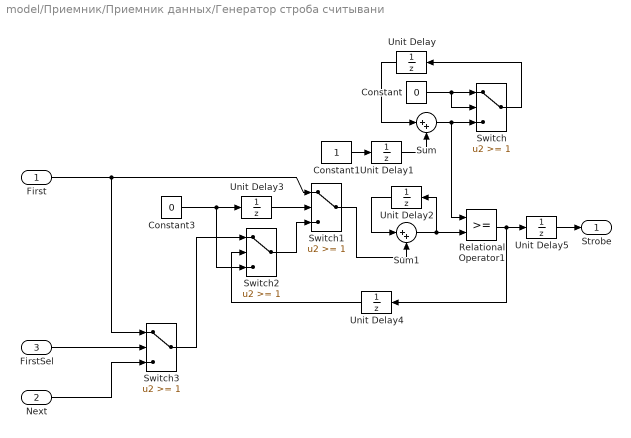
== system model/Приемник/Приемник данных/Генератор строба считывани ==
  First : Inport
  Next : Inport  Port=2
  FirstSel : Inport  Port=3
  Constant : Constant  Value=0
  Constant1 : Constant
  Constant3 : Constant  Value=0
  Relational Operator1 : RelationalOperator  RndMeth=Nearest  InputSameDT=on
  Sum : Sum  Inputs=|++  InputSameDT=on  SaturateOnIntegerOverflow=on  OutDataTypeStr=Inherit: Same as first input
  Sum1 : Sum  Inputs=|++  InputSameDT=on  SaturateOnIntegerOverflow=on  OutDataTypeStr=Inherit: Same as first input
  Switch{,1..3} (4 alike) : Switch  Threshold=1  SaturateOnIntegerOverflow=on  InputSameDT=on
  Unit Delay{,1..2,4..5} (5 alike) : UnitDelay  SampleTime=-1
  Unit Delay3 : UnitDelay  InitialCondition=1  SampleTime=-1
  Strobe : Outport
  wires:
  Sum1/1 -> Relational Operator1/2, Unit Delay2/1
  Unit Delay2/1 -> Sum1/1
  Switch1/1 -> Sum1/2
  Unit Delay3/1 -> Switch1/2
  Switch2/1 -> Switch1/3
  First/1 -> Switch1/1, Switch3/1
  Constant3/1 -> Unit Delay3/1, Switch2/3
  Relational Operator1/1 -> Unit Delay4/1, Unit Delay5/1
  Unit Delay4/1 -> Switch2/2
  Unit Delay/1 -> Sum/1
  Sum/1 -> Switch/3, Relational Operator1/1
  Constant/1 -> Switch/1, Switch/2
  Switch/1 -> Unit Delay/1
  Constant1/1 -> Unit Delay1/1
  Unit Delay1/1 -> Sum/2
  Unit Delay5/1 -> Strobe/1
  Next/1 -> Switch3/3
  Switch3/1 -> Switch2/1
  FirstSel/1 -> Switch3/2

== system model/Приемник/Приемник данных/Конвертер вектора данных в поток байтов ==
  Входной вектор : Inport
  Строб выборки : Inport  Port=2
  C3 : Constant  Value=0
  RO2 : RelationalOperator  Operator===  RndMeth=Nearest  InputSameDT=on
  SH1 : dspsigops/Sample and Hold  trig=Rising edge  initCond=0  latchinput=off
  SW3 : Switch  Threshold=1  SaturateOnIntegerOverflow=on  InputSameDT=on
  Sum1 : Sum  Inputs=|++  InputSameDT=on  SaturateOnIntegerOverflow=on  OutDataTypeStr=Inherit: Same as first input
  UD3 : UnitDelay  SampleTime=-1
  Variable Selector1 : dspindex/Variable Selector  NumInputs=1  rowsOrCols=Columns  IdxMode=Variable  Elements=[1 3]  ZerOneIdxMode=One-based  errmode=Clip Index  FillMode=on  FillValues=0
  Width1 : Width
  Выходной поток : Outport
  Размер входного вектора : Outport  Port=2
  wires:
  Входной вектор/1 -> Variable Selector1/1, Width1/1
  RO2/1 -> SW3/2
  SW3/1 -> UD3/1
  C3/1 -> SW3/1
  Sum1/1 -> SH1/1
  SH1/1 -> RO2/2, Variable Selector1/2, SW3/3
  Variable Selector1/1 -> Выходной поток/1
  Width1/1 -> RO2/1, Размер входного вектора/1
  UD3/1 -> Sum1/1
  Строб выборки/1 -> Sum1/2, SH1/Trigger

== system model/Приемник/Приемник данных/Преобразователь байт во фрейм ==
  In : Inport
  Enable : EnablePort
  Buffer : Buffer  N=pack_len  V=pack_len-1
  Frame Status Conversion3 : dspobslib/Frame Status Conversion  growRefPort=off  outframe=Sample-based
      settings: SourceProductBaseCode=DS
  Out : Outport
  wires:
  In/1 -> Buffer/1
  Buffer/1 -> Frame Status Conversion3/1
  Frame Status Conversion3/1 -> Out/1

== system model/Приемник/Приемник данных/Преобразователь бит в байты ==
  In : Inport
  Enable : EnablePort  ShowOutputPort=on
  Bit to Integer Converter : commutil2/Bit to Integer Converter  nbits=8  bitOrder=MSB first  signedOutputValues=Unsigned  outDtype=Inherit via internal rule  outDtypeSigned=Inherit via internal rule
  Buffer : Buffer  N=8  V=7
  Counter : dspswit3/Counter  Direction=Up  CountEvent=Non-zero sample  CounterSize=User defined  MaxCount=7  InitialCount=7  Output=Hit  HitValue=7  ResetInput=off  SamplesPerFrame=1  Ts=1  CntDtype=double  HitDtype=Logical
  Frame Status Conversion3 : dspobslib/Frame Status Conversion  growRefPort=off  outframe=Sample-based
      settings: SourceProductBaseCode=DS
  Out : Outport
  stb : Outport  Port=2  OutputWhenDisabled=reset  InitialOutput=[0]
  wires:
  In/1 -> Buffer/1
  Bit to Integer Converter/1 -> Frame Status Conversion3/1
  Buffer/1 -> Bit to Integer Converter/1
  Frame Status Conversion3/1 -> Out/1
  Counter/1 -> stb/1
  Enable/1 -> Counter/1

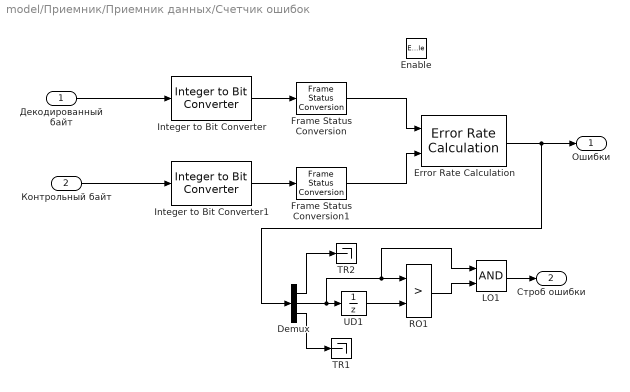
== system model/Приемник/Приемник данных/Счетчик ошибок ==
  Декодированный байт : Inport
  Контрольный байт : Inport  Port=2
  Enable : EnablePort
  Demux : Demux  Outputs=3
      settings: DisplayOption=none
  Error Rate Calculation : commsink2/Error Rate Calculation  N=0  st_delay=0  cp_mode=Entire frame  subframe=[]  PMode=Port  WsName=ErrorVec  RsMode2=off  stop=off  numErr=100  maxBits=1e6
  Frame Status Conversion : dspobslib/Frame Status Conversion  growRefPort=off  outframe=Frame-based
      settings: SourceProductBaseCode=DS
  Frame Status Conversion1 : dspobslib/Frame Status Conversion  growRefPort=off  outframe=Frame-based
      settings: SourceProductBaseCode=DS
  Integer to Bit Converter : commutil2/Integer to Bit Converter  nbits=8  signedInputValues=Unsigned  bitOrder=MSB first  outDtype=Inherit via internal rule
  Integer to Bit Converter1 : commutil2/Integer to Bit Converter  nbits=8  signedInputValues=Unsigned  bitOrder=MSB first  outDtype=Inherit via internal rule
  LO1 : Logic
  RO1 : RelationalOperator  Operator=>  RndMeth=Nearest  InputSameDT=on
  TR1 : Terminator
  TR2 : Terminator
  UD1 : UnitDelay  SampleTime=-1
  Ошибки : Outport
  Строб ошибки : Outport  Port=2  OutputWhenDisabled=reset  InitialOutput=[0]
  wires:
  Error Rate Calculation/1 -> Ошибки/1, Demux/1
  Декодированный байт/1 -> Integer to Bit Converter/1
  Контрольный байт/1 -> Integer to Bit Converter1/1
  Integer to Bit Converter/1 -> Frame Status Conversion/1
  Frame Status Conversion/1 -> Error Rate Calculation/1
  Integer to Bit Converter1/1 -> Frame Status Conversion1/1
  Frame Status Conversion1/1 -> Error Rate Calculation/2
  Demux/3 -> TR1/1
  Demux/2 -> UD1/1, RO1/1, LO1/1
  Demux/1 -> TR2/1
  UD1/1 -> RO1/2
  RO1/1 -> LO1/2
  LO1/1 -> Строб ошибки/1
